simulink model "MG_sim"  (R2020a)
settings: Solver=VariableStepAuto  StartTime=0.0  StopTime=Inf  FixedStep=N*T  RelTol=1e-3
PostLoadFcn:
  | , if any(exist('dsrtsu_mdlpostloadfcn', 'file') ~= 0), dsrtsu_mdlpostloadfcn('Execute', bdroot); end,
InitFcn:
  | , if any(exist('rtifpga_mdlclblib', 'file') ~= 0), rtifpga_mdlclblib('Init', bdroot); end,
model workspace (MAT data in the model file):
  FPGA_MG_sim_1_Register_1_1_1_write : Simulink.Signal (value not decoded)
  FPGA_MG_sim_1_Register_2_1_1_write : Simulink.Signal (value not decoded)
  FPGA_MG_sim_1_Register_3_1_1_write : Simulink.Signal (value not decoded)
values from neighbouring files (symbols this model uses):
  amp = 1    [param.m]
  fixedgain_i = 10*1000/(3*100)    (= 33.3333333333)    [param.m]    (also in params.m)
  fixedgain_vc1 = 10*10000/(3*100*2.5)    (= 133.333333333)    [param.m]
  fixedgain_vc5 = 10*22000/(3*100*2.5)    (= 293.333333333)    [param.m]
  fixedgain_vdc = 10*22000/(3*100*2.5)    (= 293.333333333)    [param.m]    (also in params.m = 586.666666667)
  freq = 50    [param.m]
  gain_iL1 = 1    [param.m]
  gain_iL2 = 1    [param.m]
  gain_iL3 = 1    [param.m]
  gain_iL4 = 1    [param.m]
  gain_vc1 = 1    [param.m]
  gain_vc5 = 1    [param.m]
  gain_vdc = 1    [param.m]    (also in params.m)
  Ii = 10    [param.m]
  Iv = 0.1    [param.m]
  Ki = 8    [param.m]
  Kp = 2.8    [param.m]
  maxd = N-1    (= 9)    [param.m]
  mind = 1    [param.m]
  N = 10    [param.m]    (also in params.m = 100)
  offset_iL1 = .2    (= 0.2)    [param.m]
  offset_iL2 = 0.2    [param.m]
  offset_iL3 = 0.3    [param.m]
  offset_iL4 = 0.25    [param.m]
  offset_vc1 = 0.27    [param.m]
  offset_vc5 = 1.3    [param.m]
  offset_vdc = 1.5    [param.m]    (also in params.m = 0)
  Pi = 0.3    [param.m]
  Pv = 0.05    [param.m]
  T = 6e-6    (= 6e-06)    [param.m]
  Tf = 1/1000    (= 0.001)    [param.m]
  Tfdc = 1/20    (= 0.05)    [param.m]
  v_dc_ref = 40    [param.m]    (also in params.m = 24)
undefined symbols (not defined in the file or in its folder): DiscIntNeverNeededParam
libraries: xbsIndex_r4 x156, rti1202lib_adc_class1 x7, rtiproclib x7, simulink x5, rti1202lib_dac_class1 x1, rtifpgainterfacelib x1
(part 2 of 5)

== system MG_sim/ESS_control ==
  v_dc : Inport
  i_bat : Inport  Port=2
  vref : Inport  Port=3
  function : TriggerPort  TriggerType=function-call  VariantControl=Variant
  Discrete PID Controller : simulink/Continuous/PID Controller  Controller=PI  Form=Parallel  TimeDomain=Discrete-time  UseExternalTs=off  SampleTime=-1  IntegratorMethod=Forward Euler  FilterMethod=Forward Euler  ControllerParametersSource=internal  P=Pv  I=Iv  D=0  UseFilter=on  N=100  TunerSelectOption=Transfer Function Based (PID Tuner App)  InitialConditionSource=internal  InitialConditionForIntegrator=0  InitialConditionForFilter=0  DifferentiatorICPrevScaledInput=0  ExternalReset=none  TrackingMode=off  Kt=1  LimitOutput=on  UpperSaturationLimit=3  LowerSaturationLimit=-5  LinearizeAsGain=off  AntiWindupMode=clamping  Kb=1  POutMin=[]  POutMax=[]  IOutMin=[]  IOutMax=[]  DOutMin=[]  DOutMax=[]  NOutMin=[]  NOutMax=[]  SumOutMin=[]  SumOutMax=[]  SaturationOutMin=[]  SaturationOutMax=[]  PParamMin=[]  PParamMax=[]  IParamMin=[]  IParamMax=[]  DParamMin=[]  DParamMax=[]  NParamMin=[]  NParamMax=[]  KbParamMin=[]  KbParamMax=[]  KtParamMin=[]  KtParamMax=[]  KbOutMin=[]  KbOutMax=[]  KtOutMin=[]  KtOutMax=[]  IntegratorOutMin=[]  IntegratorOutMax=[]  FilterOutMin=[]  FilterOutMax=[]  SumI1OutMin=[]  SumI1OutMax=[]  SumI2OutMin=[]  SumI2OutMax=[]  SumI3OutMin=[]  SumI3OutMax=[]  SumI4OutMin=[]  SumI4OutMax=[]  SumDOutMin=[]  SumDOutMax=[]  DifferentiatorOutMin=[]  DifferentiatorOutMax=[]  FilterDiffOutCoefMin=[]  FilterDiffOutCoefMax=[]  ReciprocalOutMin=[]  ReciprocalOutMax=[]  SumDenOutMin=[]  SumDenOutMax=[]  SumNumOutMin=[]  SumNumOutMax=[]  DivideOutMin=[]  DivideOutMax=[]  UdiffTsProdOutMin=[]  UdiffTsProdOutMax=[]  NTsProdOutMin=[]  NTsProdOutMax=[]  UintegralTsProdOutMin=[]  UintegralTsProdOutMax=[]  UngainTsProdOutMin=[]  UngainTsProdOutMax=[]  IntegratorContinuousStateAttributes=''  IntegratorStateMustResolveToSignalObject=off  IntegratorRTWStateStorageClass=Auto  FilterContinuousStateAttributes=''  FilterStateMustResolveToSignalObject=off  FilterRTWStateStorageClass=Auto  ParallelPVariant=InternalParameters  IdealPVariant=Disabled  IVariant=InternalParameters  DVariant=Disabled  IntegratorVariant=Discrete  SatVariant=Enabled  AWVariant=DiscClampingParallel  PCopyVariant=Disabled  TRVariant=Disabled  FdbkBlocksVariant=Forward  IdealPFdbkVariant=Disabled  SatFdbkVariant=Disabled  DerivativeFilterVariant=Disabled  NVariant=Disabled  NCopyVariant=Disabled_SignalSpec  FilterICVariant=Disabled  IntegratorICVariant=InternalICs  ExternalResetVariant=Disabled  TRSumVariant=Passthrough  SumFdbkVariant=Disabled  SumVariant=Sum_PI  TsampFilterVariant=InternalTs  TsampNgainVariant=Passthrough  TsampIntegralVariant=Passthrough
  Discrete PID Controller1 : simulink/Continuous/PID Controller  Controller=PI  Form=Parallel  TimeDomain=Discrete-time  UseExternalTs=off  SampleTime=-1  IntegratorMethod=Forward Euler  FilterMethod=Forward Euler  ControllerParametersSource=internal  P=Pi  I=Ii  D=0  UseFilter=on  N=100  TunerSelectOption=Transfer Function Based (PID Tuner App)  InitialConditionSource=internal  InitialConditionForIntegrator=0  InitialConditionForFilter=0  DifferentiatorICPrevScaledInput=0  ExternalReset=none  TrackingMode=off  Kt=1  LimitOutput=on  UpperSaturationLimit=0.97  LowerSaturationLimit=0.01  LinearizeAsGain=off  AntiWindupMode=clamping  Kb=1  POutMin=[]  POutMax=[]  IOutMin=[]  IOutMax=[]  DOutMin=[]  DOutMax=[]  NOutMin=[]  NOutMax=[]  SumOutMin=[]  SumOutMax=[]  SaturationOutMin=[]  SaturationOutMax=[]  PParamMin=[]  PParamMax=[]  IParamMin=[]  IParamMax=[]  DParamMin=[]  DParamMax=[]  NParamMin=[]  NParamMax=[]  KbParamMin=[]  KbParamMax=[]  KtParamMin=[]  KtParamMax=[]  KbOutMin=[]  KbOutMax=[]  KtOutMin=[]  KtOutMax=[]  IntegratorOutMin=[]  IntegratorOutMax=[]  FilterOutMin=[]  FilterOutMax=[]  SumI1OutMin=[]  SumI1OutMax=[]  SumI2OutMin=[]  SumI2OutMax=[]  SumI3OutMin=[]  SumI3OutMax=[]  SumI4OutMin=[]  SumI4OutMax=[]  SumDOutMin=[]  SumDOutMax=[]  DifferentiatorOutMin=[]  DifferentiatorOutMax=[]  FilterDiffOutCoefMin=[]  FilterDiffOutCoefMax=[]  ReciprocalOutMin=[]  ReciprocalOutMax=[]  SumDenOutMin=[]  SumDenOutMax=[]  SumNumOutMin=[]  SumNumOutMax=[]  DivideOutMin=[]  DivideOutMax=[]  UdiffTsProdOutMin=[]  UdiffTsProdOutMax=[]  NTsProdOutMin=[]  NTsProdOutMax=[]  UintegralTsProdOutMin=[]  UintegralTsProdOutMax=[]  UngainTsProdOutMin=[]  UngainTsProdOutMax=[]  IntegratorContinuousStateAttributes=''  IntegratorStateMustResolveToSignalObject=off  IntegratorRTWStateStorageClass=Auto  FilterContinuousStateAttributes=''  FilterStateMustResolveToSignalObject=off  FilterRTWStateStorageClass=Auto  ParallelPVariant=InternalParameters  IdealPVariant=Disabled  IVariant=InternalParameters  DVariant=Disabled  IntegratorVariant=Discrete  SatVariant=Enabled  AWVariant=DiscClampingParallel  PCopyVariant=Disabled  TRVariant=Disabled  FdbkBlocksVariant=Forward  IdealPFdbkVariant=Disabled  SatFdbkVariant=Disabled  DerivativeFilterVariant=Disabled  NVariant=Disabled  NCopyVariant=Disabled_SignalSpec  FilterICVariant=Disabled  IntegratorICVariant=InternalICs  ExternalResetVariant=Disabled  TRSumVariant=Passthrough  SumFdbkVariant=Disabled  SumVariant=Sum_PI  TsampFilterVariant=InternalTs  TsampNgainVariant=Passthrough  TsampIntegralVariant=Passthrough
  Sum : Sum  Inputs=|+-
  Sum1 : Sum  Inputs=|+-
  y1 : Outport
  wires:
  vref/1 -> Sum/1
  Sum1/1 -> Discrete PID Controller1/1
  Sum/1 -> Discrete PID Controller/1
  v_dc/1 -> Sum/2
  Discrete PID Controller1/1 -> y1/1
  i_bat/1 -> Sum1/2
  Discrete PID Controller/1 -> Sum1/1

== system MG_sim/MPPT_system ==
  v_PV : Inport
  i_PV : Inport  Port=2
  v_DC : Inport  Port=3
  function : TriggerPort  TriggerType=function-call  VariantControl=Variant
  MATLAB Function : MATLAB Function  TreatAsAtomicUnit=on
  Terminator : Terminator
  Terminator1 : Terminator
  d : Outport
  wires:
  MATLAB Function/2(d) -> d/1
  i_PV/1 -> MATLAB Function/2(i)
  MATLAB Function/1(v_PandO) -> Terminator/1
  v_PV/1 -> MATLAB Function/1(v_pv)
  v_DC/1 -> MATLAB Function/3(v_dc)
  MATLAB Function/3(P) -> Terminator1/1

== system MG_sim/RTI Data ==
  RTI Data Store : Subsystem  Tag="struct('public',struct('sub',struct('name',{{'MG_sim'}},'data',{{struct('TH',struct('thTaskInfo',struct('taskType',{'TIMER','HWINT','TMRINT','SWINT','GLINT'},'tasksNumOf',{1,3,0,0,0},'srcIds',{{'TIMERA'},{'FPGACL1FPGA_INTP0Ch1','FPGACL1FPGA_INTP0Ch2','FPGACL1FPGA_INTP0Ch0'},{},{},{}},'taskNames',{{['Timer Task 1']},{'PROC_INT_BL1',['PROC_INT_BL1 - interr'],['PROC_INT_BL1 - interr1']},{},{},{}})),'th_tc',struct('dataType',{'TASK','TASK','TASK','TASK'},'taskGroupId',{'','','',''},'taskGroupList',{{},{},{},{}},'taskSchedulingPolicy',{'FCFS','FCFS','FCFS','FCFS'},'taskType',{'TIMER','HWINT','HWINT','HWINT'},'blkh',{-1,['MG_sim/PROC_INT_BL1/Common Hardware' char(10) 'Interrupt Interface'],['MG_sim/PROC_INT_BL1 - interr/Common Hardware' char(10) 'Interrupt Interface'],['MG_sim/PROC_INT_BL1 - interr1/Common Hardware' char(10) 'Interrupt Interface']},'srcId',{'TIMERA','FPGACL1FPGA_INTP0Ch1','FPGACL1FPGA_INTP0Ch2','FPGACL1FPGA_INTP0Ch0'},'srcSgnName',{['Timer A interrupt'],['FPGA Type CL1 FPGA_INT Port 0 Channel 1'],['FPGA Type CL1 FPGA_INT Port 0 Channel 2'],['FPGA Type CL1 FPGA_INT Port 0 Channel 0']},'srcCpuName',{'','','',''},'taskName',{['Timer Task 1  [6e-05] s'],'PROC_INT_BL1',['PROC_INT_BL1 - interr'],['PROC_INT_BL1 - interr1']},'taskNameDisplayExt',{'','','',''},'smplTime',{6e-5,0,0,0},'smplTimeOffs',{0,0,0,0},'hasFixedPriority',{0,0,0,0},'priority',{1,2,3,4},'hasFixedOvc',{0,0,0,0},'ovcType',{1,1,1,1},'ovcMax',{1,1,1,1}),'tc_th',struct('dataType',{'TASK','TASK','TASK','TASK'},'taskGroupId',{'','','',''},'taskGroupList',{{},{},{},{}},'taskSchedulingPolicy',{'FCFS','FCFS','FCFS','FCFS'},'taskType',{'TIMER','HWINT','HWINT','HWINT'},'blkh',{-1,['MG_sim/PROC_INT_BL1/Common Hardware' char(10) 'Interrupt Interface'],['MG_sim/PROC_INT_BL1 - interr/Common Hardware' char(10) 'Interrupt Interface'],['MG_sim/PROC_INT_BL1 - interr1/Common Hardware' char(10) 'Interrupt Interface']},'srcId',{'TIMERA','FPGACL1FPGA_INTP0Ch1','FPGACL1FPGA_INTP0Ch2','FPGACL1FPGA_INTP0Ch0'},'srcSgnName',{['Timer A interrupt'],['FPGA Type CL1 FPGA_INT Port 0 Channel 1'],['FPGA Type CL1 FPGA_INT Port 0 Channel 2'],['FPGA Type CL1 FPGA_INT Port 0 Channel 0']},'srcCpuName',{'','','',''},'taskName',{['Timer Task 1  [6e-05] s'],'PROC_INT_BL1',['PROC_INT_BL1 - interr'],['PROC_INT_BL1 - interr1']},'taskNameDisplayExt',{'','','',''},'smplTime',{6e-5,0,0,0},'smplTimeOffs',{0,0,0,0},'hasFixedPriority',{0,0,0,0},'priority',{1,2,3,4},'hasFixedOvc',{0,0,0,0},'ovcType',{1,1,1,1},'ovcMax',{1,1,1,1}))}})),'private',struct('version',struct('dsVer',uint32(2)),'access',struct('modified',['11-Apr-2025 21:33:23'],'type','Model','isPerm',1)))"  mask(RTI_DATA_STORE){}
      mask help:
      | RTI Data Store Block. This block is used by RTI to store internal model dependent data. Deleting this block will result in data loss.
      |
      | NEVER DELETE, COPY, OR MODIFY THIS BLOCK!
      mask Help:
      | RTI Data Store Block. This block is used by RTI to store internal model dependent data. Deleting this block will result in data loss.
      | 
      | NEVER DELETE, COPY, OR MODIFY THIS BLOCK!
      mask Display: text(0.5, 0.5, ' ', 'HorizontalAlignment', 'center');

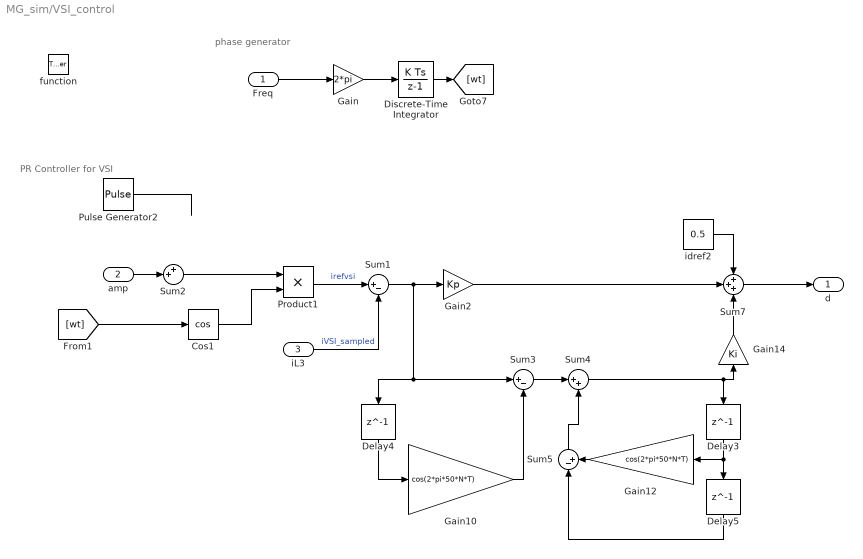
== system MG_sim/VSI_control ==
  note: phase generator
  note: PR Controller for VSI
  Freq : Inport
  amp : Inport  Port=2
  iL3 : Inport  Port=3
  function : TriggerPort  TriggerType=function-call  VariantControl=Variant
  Cos1 : Trigonometry  Operator=cos
  Delay3 : Delay  DelayLength=1
  Delay4 : Delay  DelayLength=1
  Delay5 : Delay  DelayLength=1
  Discrete-Time Integrator : DiscreteIntegrator  SampleTime=-1  ICPrevOutput=DiscIntNeverNeededParam  ICPrevScaledInput=DiscIntNeverNeededParam
  Gain : Gain  Gain=2*pi
  Gain10 : Gain  Gain=cos(2*pi*50*N*T)
  Gain12 : Gain  Gain=cos(2*pi*50*N*T)
  Gain14 : Gain  Gain=Ki
  Gain2 : Gain  Gain=Kp
  Product1 : Product
  Pulse Generator2 : DiscretePulseGenerator  Amplitude=0.5  Period=5000  PulseWidth=2500  SampleTime=-1
  Sum1 : Sum  Inputs=|+-
  Sum2 : Sum  Inputs=++|
  Sum3 : Sum  Inputs=|+-
  Sum4 : Sum  Inputs=|++
  Sum5 : Sum  Inputs=|-+
  Sum7 : Sum  Inputs=+++
  idref2 : Constant  Value=0.5
  d : Outport
  wires:
  Freq/1 -> Gain/1
  Discrete-Time Integrator/1 -> [wt]
  Gain/1 -> Discrete-Time Integrator/1
  Gain14/1 -> Sum7/3
  idref2/1 -> Sum7/1
  iL3/1 -> Sum1/2  "iVSI_sampled"
  Gain2/1 -> Sum7/2
  Gain10/1 -> Sum3/2
  Delay4/1 -> Gain10/1
  Sum1/1 -> Gain2/1, Delay4/1, Sum3/1
  Delay3/1 -> Gain12/1, Delay5/1
  Delay5/1 -> Sum5/1
  Pulse Generator2/1 -> ?
  Product1/1 -> Sum1/1  "irefvsi"
  Sum2/1 -> Product1/1
  [wt] -> Cos1/1
  Sum5/1 -> Sum4/2
  Sum3/1 -> Sum4/1
  Gain12/1 -> Sum5/2
  Cos1/1 -> Product1/2
  Sum4/1 -> Delay3/1, Gain14/1
  amp/1 -> Sum2/2
  Sum7/1 -> d/1
